simulink model "twowithout1"  (R2014b)
settings: Solver=ode45  SolverMode=SingleTasking  StartTime=0.0  StopTime=10.0  RelTol=1e-3
settings Model: CovMetricSettings=dwe  CovHtmlReporting=off  covSaveCumulativeToWorkspaceVar=off  CovSaveSingleToWorkspaceVar=off  CovExternalEMLEnable=on  CovSFcnEnable=on  Creator=HEISENBERG  LastModifiedBy=HEISENBERG
settings DataIOCC: LimitDataPoints=off  SaveFormat=StructureWithTime  ReturnWorkspaceOutputs=on
settings DebuggingCC: SolverPrmCheckMsg=none  UnconnectedInputMsg=none  UnconnectedOutputMsg=none  UnconnectedLineMsg=none  FrameProcessingCompatibilityMsg=error  SFUnexpectedBacktrackingDiag=error  SFNoUnconditionalDefaultTransitionDiag=error
settings HardwareCC: ProdBitPerPointer=64  ProdLargestAtomicFloat=Float  ProdIntDivRoundTo=Zero  ProdEndianess=LittleEndian  ProdHWDeviceType=Specified
settings ModelReferenceCC: PropagateSignalLabelsOutOfModel=on
settings SFSimCC: SimUseLocalCustomCode=on
settings RTWCC: RTWUseLocalCustomCode=on
settings GRTTargetCC: TargetLangStandard=C99 (ISO)

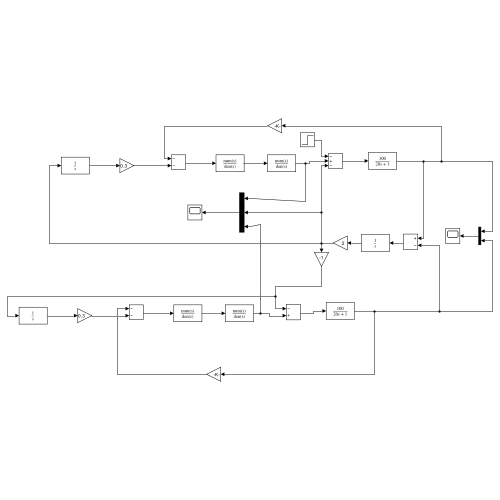
[thumbnail: Simulink's stored preview of the top-level diagram]
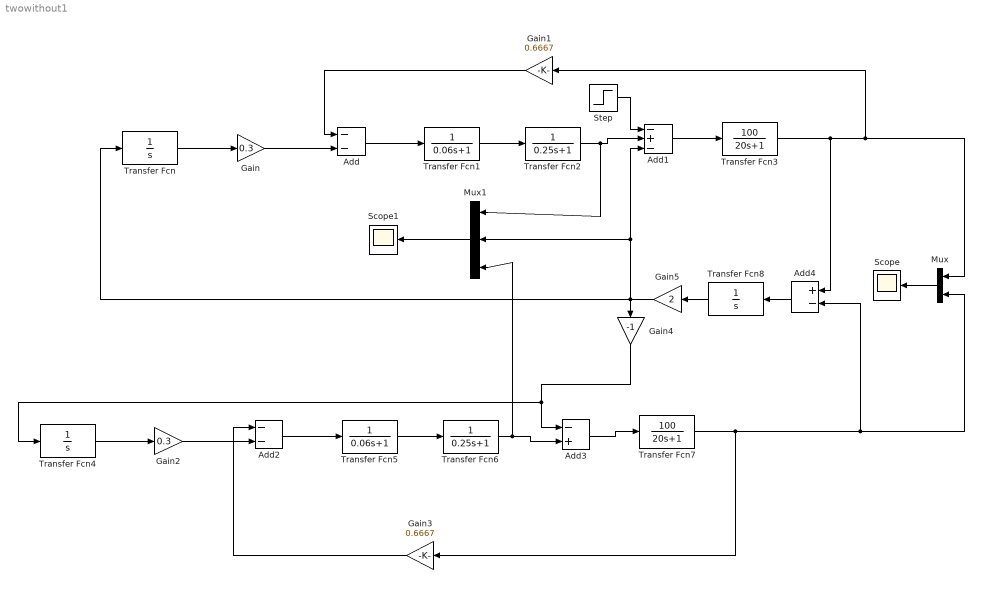
== system twowithout1 ==
  Add : Sum  Inputs=--
  Add1 : Sum  Inputs=-+-
  Add2 : Sum  Inputs=--
  Add3 : Sum  Inputs=-+
  Add4 : Sum  Inputs=+-
  Gain : Gain  Gain=0.3
  Gain1 : Gain  Gain=0.6667
  Gain2 : Gain  Gain=0.3
  Gain3 : Gain  Gain=0.6667
  Gain4 : Gain  Gain=-1
  Gain5 : Gain  Gain=2
  Mux : Mux  Inputs=2
  Mux1 : Mux  Inputs=3
  Scope : Scope
      settings: TimeRange=auto  MaxDataPoints=5000  SaveToWorkspace=off  SaveName=ScopeData  YMin=-1.47881  YMax=0.16431  SampleTime=-1
  Scope1 : Scope
      settings: TimeRange=auto  MaxDataPoints=5000  SaveToWorkspace=off  YMin=-0.9463  YMax=1.18528  SampleTime=-1
  Step : Step  SampleTime=0
  Transfer Fcn : TransferFcn  Denominator=[1 0]
  Transfer Fcn1 : TransferFcn  Denominator=[0.06 1]
  Transfer Fcn2 : TransferFcn  Denominator=[0.25 1]
  Transfer Fcn3 : TransferFcn  Numerator=[100]  Denominator=[20 1]
  Transfer Fcn4 : TransferFcn  Denominator=[1 0]
  Transfer Fcn5 : TransferFcn  Denominator=[0.06 1]
  Transfer Fcn6 : TransferFcn  Denominator=[0.25 1]
  Transfer Fcn7 : TransferFcn  Numerator=[100]  Denominator=[20 1]
  Transfer Fcn8 : TransferFcn  Denominator=[1 0]
  wires:
  Transfer Fcn/1 -> Gain/1
  Gain/1 -> Add/2
  Add/1 -> Transfer Fcn1/1
  Transfer Fcn1/1 -> Transfer Fcn2/1
  Transfer Fcn2/1 -> Mux1/1, Add1/2
  Add1/1 -> Transfer Fcn3/1
  Transfer Fcn3/1 -> Add4/1, Mux/1, Gain1/1
  Gain1/1 -> Add/1
  Mux/1 -> Scope/1
  Transfer Fcn7/1 -> Add4/2, Mux/2, Gain3/1
  Gain2/1 -> Add2/2
  Transfer Fcn5/1 -> Transfer Fcn6/1
  Add2/1 -> Transfer Fcn5/1
  Add3/1 -> Transfer Fcn7/1
  Transfer Fcn4/1 -> Gain2/1
  Transfer Fcn6/1 -> Mux1/3, Add3/2
  Gain3/1 -> Add2/1
  Mux1/1 -> Scope1/1
  Gain5/1 -> Transfer Fcn/1, Gain4/1, Mux1/2, Add1/3
  Transfer Fcn8/1 -> Gain5/1
  Gain4/1 -> Transfer Fcn4/1, Add3/1
  Step/1 -> Add1/1
  Add4/1 -> Transfer Fcn8/1
